simulink model "EarlyReturn20_2018a"  (R2018a)
settings: Solver=VariableStepAuto  StartTime=0.0  StopTime=0.1  RelTol=1e-3
settings Model: Creator=BEAR  LastModifiedBy=bzhan

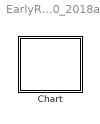
== system EarlyReturn20_2018a ==
  Chart : Stateflow chart  TreatAsAtomicUnit=on

== stateflow chart EarlyReturn20_2018a/Chart ==
  settings: updateMethod=DISCRETE  sampleTime=0.1
  state S
    en: f("enS")
    du: f("duS")
    ex: f("exS")
    state A1
    state A2
    (junction 15) -> A2 : {f("ca2")}/{f("ta2")}
    A1 -> (junction 15) : {f("ca1")}/{E;f("ta1")}
    (default) -> A1
  state T
    en: f("enT")
  (default) -> S
  S -> T : E
  data: s function_input
  events: E local FUNCTION_CALL_EVENT
  function f(s):
    | function f(s)
    |   fprintf(s+"\n");
